simulink library "Heat_Capacity"  (R2018b)
settings: Solver=ode45  StartTime=0.0  StopTime=10.0  RelTol=1e-3  EnableMultiTasking=on
undefined symbols (not defined in the file): CarnotCallbacks_Heat_Capacity
settings Model: Creator=lena.frank  LastModifiedBy=P41573
settings DataIOCC: LimitDataPoints=on  SaveFormat=Array  SignalLoggingSaveFormat=ModelDataLogs
settings OptimizationCC: ExpressionDepthLimit=2147483647  LifeSpan=inf
settings DebuggingCC: UnderspecifiedInitializationDetection=Classic  MergeDetectMultiDrivingBlocksExec=none  SolverPrmCheckMsg=warning  FcnCallInpInsideContextMsg=warning  StateNameClashWarn=warning  SFUnexpectedBacktrackingDiag=warning  SFNoUnconditionalDefaultTransitionDiag=warning  SFExecutionAtInitializationDiag=none
settings HardwareCC: ProdBitPerPointer=32  ProdBitPerSizeT=32  ProdBitPerPtrDiffT=32  ProdLargestAtomicFloat=None  ProdIntDivRoundTo=Undefined  ProdEndianess=Unspecified  ProdWordSize=32  ProdHWDeviceType=32-bit Generic
settings ModelReferenceCC: PropagateSignalLabelsOutOfModel=off
settings SFSimCC: SimUseLocalCustomCode=off
settings RTWCC: RTWUseLocalCustomCode=off
settings CodeAppCC: StateflowObjectComments=on
settings GRTTargetCC: TargetLangStandard=C89/C90 (ANSI)  GeneratePreprocessorConditionals=Disable all  CombineOutputUpdateFcns=off  GRTInterface=on
settings ConfigComp: CovMetricSettings=dw  CovHtmlReporting=on  CovSaveCumulativeToWorkspaceVar=on  CovSaveSingleToWorkspaceVar=on  CovExternalEMLEnable=off

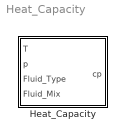
== system Heat_Capacity ==
  Heat_Capacity : Subsystem  LoadFcn=CarnotCallbacks_Heat_Capacity('LoadFcn');  InitFcn=load('THB.mat');  VariantControl=CarlibClassic  mask(heat capacity){INPUTARGUMENTS=state variables (classic), DEBUGLEVEL=DEBUGLEVEL, MAXTOTALWARNINGS=inf, MAXCONSECUTIVEWARNINGS=inf, WRITETOFILE=0, FILENAME='errors.txt'}
      mask prompts: INPUTARGUMENTS "Input arguments"; DEBUGLEVEL "Debug level"; MAXTOTALWARNINGS "maximum number of total warning"; MAXCONSECUTIVEWARNINGS "maximum number of consecutive warnings"; WRITETOFILE "write messages to file"; FILENAME "filename for error messages"
      mask help:
      | Calculates the  heat_capacity of fluids [J/(kg*K)]. Calls calls the function "heat_capacity" in the CARNOT library "carlib".
      | You may use the block "GlobalMessageLevel" in the Toolbox to handle the debugging messages.
      | FluidType        Remarks
      | 1: water          fluid mix is vapourcontent in the 2-phase region
      | 2: air              fluid mix is (kg water) / (kg dry air)
      | 3: cotton oil       -
      | 4: silicone oil     -
      | 5: water-glycol   fluid mix is volume partition [0..1] of propylen glycol
      | 6: Tyfocor LS     function only available in liquid phase
      | 7: Water Constant = 4181.0 J/kg/K (water at 20°C)
      | 8: Air Constant   = 1007.0 J/kg/K (air at 20°C)
      mask init:
      | %Inports
      | CarnotCallbacks_Heat_Capacity('CreateInports');
      | 
      | %global debug level
      | [DEBUGLEVEL, MAXTOTALWARNINGS, MAXCONSECUTIVEWARNINGS, WRITETOFILE, FILENAME] = CarnotCallbacks_Heat_Capacity('CheckDebugLevels', DEBUGLEVEL, MAXTOTALWARNINGS, MAXCONSECUTIVEWARNINGS, WRITETOFILE, FILENAME);
      mask Help: web(fullfile(path_carnot('help'),'heat_capacity_mdl.html'),'-helpbrowser')
      mask TypeOptions INPUTARGUMENTS: state variables (classic) | THB | THV
      mask Callback INPUTARGUMENTS: CarnotCallbacks_Heat_Capacity('MaskVisibilities');
      mask TypeOptions DEBUGLEVEL: DEBUGLEVEL | INFOLEVEL | WARNINGLEVEL | ERRORLEVEL | FATALLEVEL | NOLEVEL
      mask DialogControl ParameterTabVar0 Prompt: Parameters
      mask DialogControl ParameterTabVar01 Prompt: Debugging

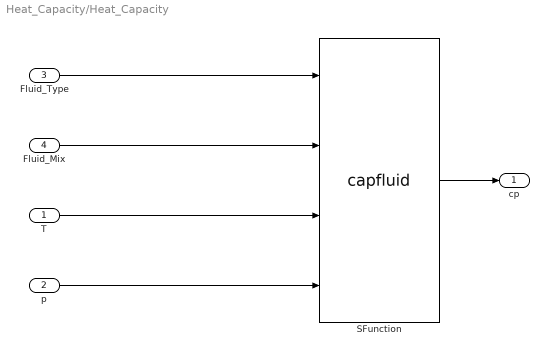
== system Heat_Capacity/Heat_Capacity ==
  T : Inport
  p : Inport  Port=2
  Fluid_Type : Inport  Port=3
  Fluid_Mix : Inport  Port=4
  SFunction : S-Function  FunctionName=capfluid  Parameters=DEBUGLEVEL-1,MAXTOTALWARNINGS,MAXCONSECUTIVEWARNINGS,WRITETOFILE,FILENAME  SFunctionDeploymentMode=off  EnableBusSupport=off
  cp : Outport
  wires:
  SFunction/1 -> cp/1
  T/1 -> SFunction/3
  p/1 -> SFunction/4
  Fluid_Type/1 -> SFunction/1
  Fluid_Mix/1 -> SFunction/2
